simulink model "Boost_Non_Ideal_Non_Linear_Model"  (R2022b)
settings: Solver=VariableStepAuto  StartTime=0.0  StopTime=0.02  RelTol=1e-3
values from neighbouring files (symbols this model uses):
  C = 1e-3    (= 0.001)    [Boost_Converter_Parameters.m]
  Dnom = 0.55    [Boost_Converter_Parameters.m]
  fS = 10^5    (= 100000)    [Boost_Converter_Parameters.m]
  L = 100e-6    (= 0.0001)    [Boost_Converter_Parameters.m]
  rC = 0.01    [Boost_Converter_Parameters.m]
  rDS = 0.055    [Boost_Converter_Parameters.m]
  RF = 0.01    [Boost_Converter_Parameters.m]
  rL = 0.08    [Boost_Converter_Parameters.m]
  RL = 4.5    [Boost_Converter_Parameters.m]
  VF = 0.7    [Boost_Converter_Parameters.m]
  Vinnom = 24    [Boost_Converter_Parameters.m]
settings Model: Creator=YESHIWAS  LastModifiedBy=YESHIWAS
settings DataIOCC: ReturnWorkspaceOutputs=off

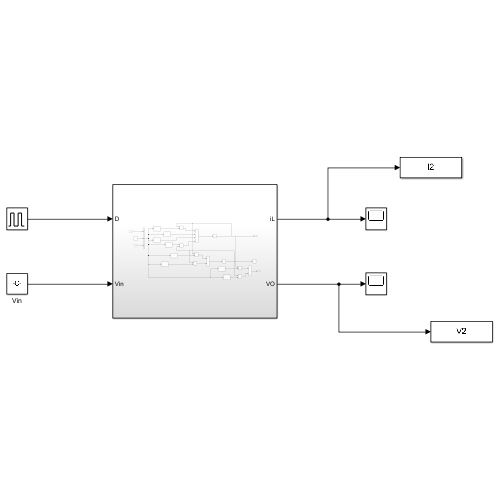
[thumbnail: Simulink's stored preview of the top-level diagram]
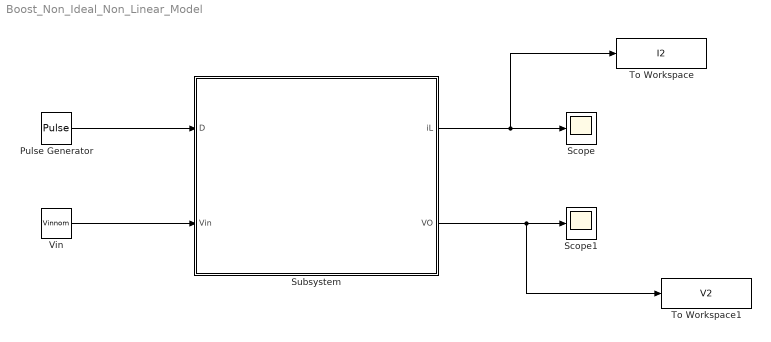
== system Boost_Non_Ideal_Non_Linear_Model ==
  Pulse Generator : DiscretePulseGenerator  PulseType=Time based  Period=1/fS  PulseWidth=Dnom*100
  Scope : Scope
  Scope1 : Scope
  Subsystem : Subsystem
  To Workspace : ToWorkspace  VariableName=I2  SaveFormat=Structure With Time  SampleTime=-1
  To Workspace1 : ToWorkspace  VariableName=V2  SaveFormat=Structure With Time  SampleTime=-1
  Vin : Constant  Value=Vinnom
  wires:
  Pulse Generator/1 -> Subsystem/1(D)
  Vin/1 -> Subsystem/2(Vin)
  Subsystem/2(VO) -> To Workspace1/1, Scope1/1
  Subsystem/1(iL) -> To Workspace/1, Scope/1

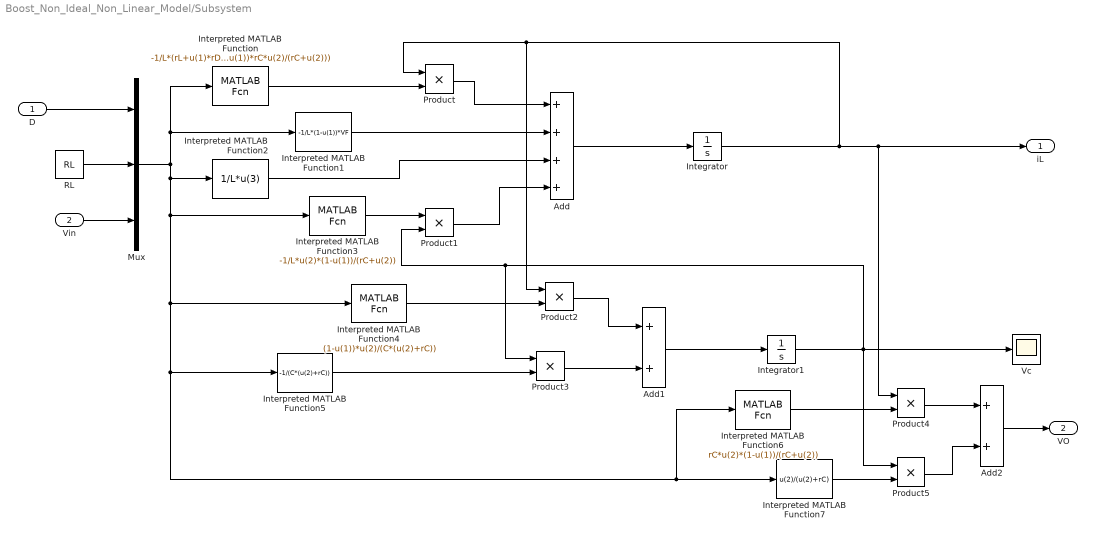
== system Boost_Non_Ideal_Non_Linear_Model/Subsystem ==
  D : Inport
  Vin : Inport  Port=2
  Add : Sum  Inputs=++++
  Add1 : Sum
  Add2 : Sum
  Integrator : Integrator
  Integrator1 : Integrator
  Interpreted MATLAB Function : MATLABFcn  MATLABFcn=-1/L*(rL+u(1)*rDS+(1-u(1))*RF+(1-u(1))*rC*u(2)/(rC+u(2)))
  Interpreted MATLAB Function1 : MATLABFcn  MATLABFcn=-1/L*(1-u(1))*VF
  Interpreted MATLAB Function2 : MATLABFcn  MATLABFcn=1/L*u(3)
  Interpreted MATLAB Function3 : MATLABFcn  MATLABFcn=-1/L*u(2)*(1-u(1))/(rC+u(2))
  Interpreted MATLAB Function4 : MATLABFcn  MATLABFcn=(1-u(1))*u(2)/(C*(u(2)+rC))
  Interpreted MATLAB Function5 : MATLABFcn  MATLABFcn=-1/(C*(u(2)+rC))
  Interpreted MATLAB Function6 : MATLABFcn  MATLABFcn=rC*u(2)*(1-u(1))/(rC+u(2))
  Interpreted MATLAB Function7 : MATLABFcn  MATLABFcn=u(2)/(u(2)+rC)
  Mux : Mux  Inputs=3
  Product{,1..5} (6 alike) : Product
  RL : Constant  Value=RL
  Vc : Scope
  iL : Outport
  VO : Outport  Port=2
  wires:
  Integrator/1 -> Product4/1, iL/1, Product2/1, Product/1
  Add/1 -> Integrator/1
  Add1/1 -> Integrator1/1
  Interpreted MATLAB Function/1 -> Product/2
  Interpreted MATLAB Function3/1 -> Product1/1
  Product/1 -> Add/1
  Interpreted MATLAB Function1/1 -> Add/2
  Interpreted MATLAB Function2/1 -> Add/3
  Product1/1 -> Add/4
  Mux/1 -> Interpreted MATLAB Function1/1, Interpreted MATLAB Function/1, Interpreted MATLAB Function2/1, Interpreted MATLAB Function3/1, Interpreted MATLAB Function4/1, Interpreted MATLAB Function5/1, Interpreted MATLAB Function7/1, Interpreted MATLAB Function6/1
  Interpreted MATLAB Function4/1 -> Product2/2
  Interpreted MATLAB Function5/1 -> Product3/2
  Product3/1 -> Add1/2
  Product2/1 -> Add1/1
  D/1 -> Mux/1
  RL/1 -> Mux/2
  Vin/1 -> Mux/3
  Interpreted MATLAB Function7/1 -> Product5/2
  Integrator1/1 -> Vc/1, Product5/1, Product3/1, Product1/2
  Interpreted MATLAB Function6/1 -> Product4/2
  Product4/1 -> Add2/1
  Product5/1 -> Add2/2
  Add2/1 -> VO/1
